simulink model "test_com_PowerLimitation"  (R2017a)
settings: Solver=FixedStepDiscrete  StartTime=0.0  StopTime=10  FixedStep=0.001  RelTol=1e-3
settings Model: DataDictionary=controller_dict.sldd  Creator=rieth  LastModifiedBy=rieth
settings OptimizationCC: UseDivisionForNetSlopeComputation=on

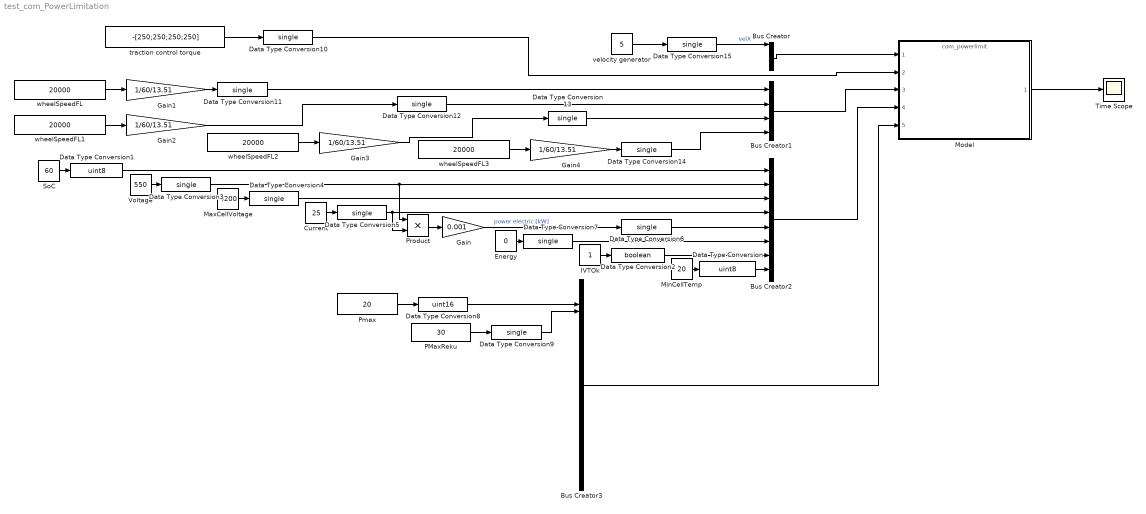
== system test_com_PowerLimitation ==
  Bus Creator : BusCreator  Inputs=8  OutDataTypeStr=Bus: control_VehicleStateRB
  Bus Creator1 : BusCreator  Inputs=4  OutDataTypeStr=Bus: control_WheelSpeed
  Bus Creator2 : BusCreator  Inputs=8  OutDataTypeStr=Bus: control_Electric
  Bus Creator3 : BusCreator  Inputs=28  OutDataTypeStr=Bus: control_Settings
  Current : Constant  Value=25
  Data Type Conversion : DataTypeConversion  OutDataTypeStr=uint8
  Data Type Conversion1 : DataTypeConversion  OutDataTypeStr=uint8
  Data Type Conversion{3..7,9..15} (12 alike) : DataTypeConversion  OutDataTypeStr=single
  Data Type Conversion2 : DataTypeConversion  OutDataTypeStr=boolean
  Data Type Conversion8 : DataTypeConversion  OutDataTypeStr=uint16
  Energy : Constant  Value=0
  Gain : Gain  Gain=0.001
  Gain{1..4} (4 alike) : Gain  Gain=1/60/13.51
  IVTOk : Constant
  MaxCellVoltage : Constant  Value=4200
  MinCellTemp : Constant  Value=20
  Model : ModelReference  ModelNameDialog=com_powerlimit  SimulationMode=Normal  ModelReferenceVersion=1.91
  PMaxReku : Constant  Value=30
  Pmax : Constant  Value=20
  Product : Product
  SoC : Constant  Value=60
  Time Scope : Scope
  Voltage : Constant  Value=550
  traction control torque : Constant  Value=-[250;250;250;250]
  velocity generator : Constant  Value=5
  wheelSpeedFL{,1..3} (4 alike) : Constant  Value=20000
  wires:
  Model/1 -> Time Scope/1
  velocity generator/1 -> Data Type Conversion15/1
  Bus Creator/1 -> Model/1
  traction control torque/1 -> Data Type Conversion10/1
  wheelSpeedFL/1 -> Gain1/1
  Bus Creator1/1 -> Model/3
  Gain2/1 -> Data Type Conversion12/1
  Gain3/1 -> Data Type Conversion13/1
  Gain4/1 -> Data Type Conversion14/1
  Bus Creator2/1 -> Model/4
  SoC/1 -> Data Type Conversion1/1
  Voltage/1 -> Data Type Conversion3/1
  MaxCellVoltage/1 -> Data Type Conversion4/1
  Current/1 -> Data Type Conversion5/1
  Product/1 -> Gain/1
  Energy/1 -> Data Type Conversion7/1
  IVTOk/1 -> Data Type Conversion2/1
  MinCellTemp/1 -> Data Type Conversion/1
  Data Type Conversion/1 -> Bus Creator2/8
  Data Type Conversion1/1 -> Bus Creator2/1
  Data Type Conversion2/1 -> Bus Creator2/7
  Data Type Conversion3/1 -> Product/1, Bus Creator2/2
  Data Type Conversion4/1 -> Bus Creator2/3
  Data Type Conversion5/1 -> Product/2, Bus Creator2/4
  Data Type Conversion6/1 -> Bus Creator2/5
  Data Type Conversion7/1 -> Bus Creator2/6
  Pmax/1 -> Data Type Conversion8/1
  PMaxReku/1 -> Data Type Conversion9/1
  Data Type Conversion8/1 -> Bus Creator3/3
  Data Type Conversion9/1 -> Bus Creator3/4
  Data Type Conversion10/1 -> Model/2
  Bus Creator3/1 -> Model/5
  Data Type Conversion11/1 -> Bus Creator1/1
  Data Type Conversion12/1 -> Bus Creator1/2
  Data Type Conversion13/1 -> Bus Creator1/3
  Data Type Conversion14/1 -> Bus Creator1/4
  Data Type Conversion15/1 -> Bus Creator/1  "velX"
  Gain/1 -> Data Type Conversion6/1  "power electric [kW]"
  Gain1/1 -> Data Type Conversion11/1
  wheelSpeedFL1/1 -> Gain2/1
  wheelSpeedFL2/1 -> Gain3/1
  wheelSpeedFL3/1 -> Gain4/1
